simulink model "simulink_model_pid_controller_IT2_controller_ds"  (R2022b)
settings: Solver=VariableStepAuto  StartTime=0.0  StopTime=1  RelTol=1e-3
libraries: slpidlib x1
settings Model: Creator=giris  LastModifiedBy=giris

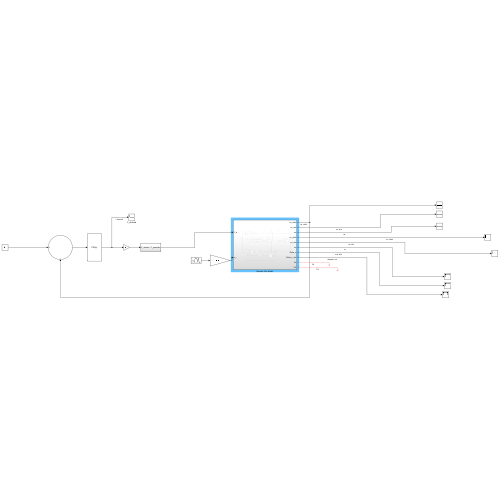
[thumbnail: Simulink's stored preview of the top-level diagram]
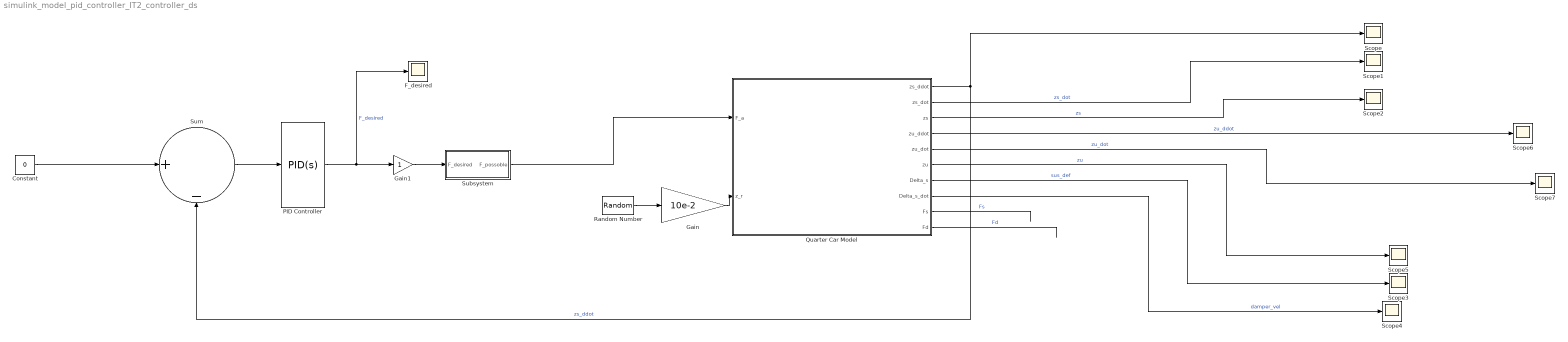
== system simulink_model_pid_controller_IT2_controller_ds ==
  Constant : Constant  Value=0
  F_desired : Scope
  Gain : Gain  Gain=10e-2
  Gain1 : Gain
  PID Controller : slpidlib/PID Controller  Controller=PID  Form=Parallel  TimeDomain=Continuous-time  UseExternalTs=off  SampleTime=-1  IntegratorMethod=Forward Euler  FilterMethod=Forward Euler  ControllerParametersSource=internal  P=8000  I=500  UseKiTs=off  D=400  N=100  UseFilter=on  TunerSelectOption=Transfer Function Based (PID Tuner App)  InitialConditionSource=internal  InitialConditionForIntegrator=0  InitialConditionForFilter=0  DifferentiatorICPrevScaledInput=0  ExternalReset=none  TrackingMode=off  Kt=1  LimitOutput=off  SatLimitsSource=internal  UpperSaturationLimit=inf  LowerSaturationLimit=-inf  LinearizeAsGain=on  AntiWindupMode=none  Kb=1  LimitIntegrator=off  UpperIntegratorSaturationLimit=inf  LowerIntegratorSaturationLimit=-inf  POutMin=[]  POutMax=[]  IOutMin=[]  IOutMax=[]  DOutMin=[]  DOutMax=[]  NOutMin=[]  NOutMax=[]  SumOutMin=[]  SumOutMax=[]  SaturationOutMin=[]  SaturationOutMax=[]  PParamMin=[]  PParamMax=[]  IParamMin=[]  IParamMax=[]  DParamMin=[]  DParamMax=[]  NParamMin=[]  NParamMax=[]  KbParamMin=[]  KbParamMax=[]  KtParamMin=[]  KtParamMax=[]  KbOutMin=[]  KbOutMax=[]  KtOutMin=[]  KtOutMax=[]  IntegratorOutMin=[]  IntegratorOutMax=[]  FilterOutMin=[]  FilterOutMax=[]  SumI1OutMin=[]  SumI1OutMax=[]  SumI2OutMin=[]  SumI2OutMax=[]  SumI3OutMin=[]  SumI3OutMax=[]  SumI4OutMin=[]  SumI4OutMax=[]  SumDOutMin=[]  SumDOutMax=[]  DifferentiatorOutMin=[]  DifferentiatorOutMax=[]  FilterDiffOutCoefMin=[]  FilterDiffOutCoefMax=[]  ReciprocalOutMin=[]  ReciprocalOutMax=[]  SumDenOutMin=[]  SumDenOutMax=[]  SumNumOutMin=[]  SumNumOutMax=[]  DivideOutMin=[]  DivideOutMax=[]  UdiffTsProdOutMin=[]  UdiffTsProdOutMax=[]  NTsProdOutMin=[]  NTsProdOutMax=[]  UintegralTsProdOutMin=[]  UintegralTsProdOutMax=[]  UngainTsProdOutMin=[]  UngainTsProdOutMax=[]  ClampingZeroOutDataTypeStr=Inherit: Inherit via back propagation  ClampingZeroOutMin=[]  ClampingZeroOutMax=[]  FilterDenConstantOutDataTypeStr=Inherit: Inherit via back propagation  FilterDenConstantOutMin=[]  FilterDenConstantOutMax=[]  PCopyOutDataTypeStr=Inherit: Inherit via back propagation  PCopyOutMin=[]  PCopyOutMax=[]  NCopyOutDataTypeStr=Inherit: Inherit via back propagation  NCopyOutMin=[]  NCopyOutMax=[]  IntegratorContinuousStateAttributes=''  IntegratorStateMustResolveToSignalObject=off  IntegratorRTWStateStorageClass=Auto  FilterContinuousStateAttributes=''  FilterStateMustResolveToSignalObject=off  FilterRTWStateStorageClass=Auto  ParallelPVariant=InternalParameters  IdealPVariant=Disabled  IVariant=InternalParameters  DVariant=InternalParameters  IntegratorVariant=Continuous  SatVariant=Disabled  AWVariant=Passthrough  PCopyVariant=Disabled  TRVariant=Disabled  FdbkBlocksVariant=Forward  IdealPFdbkVariant=Disabled  SatFdbkVariant=Disabled  DerivativeFilterVariant=ContFilter  NVariant=InternalParameters  NCopyVariant=Disabled  FilterICVariant=InternalICsFilter  IntegratorICVariant=InternalICs  ExternalResetVariant=Disabled  TRSumVariant=Passthrough  SumFdbkVariant=Disabled  SumVariant=Sum_PID  TsampFilterVariant=InternalTs  TsampNgainVariant=Passthrough  TsampIntegralVariant=Passthrough  ExternalSaturationOutDataTypeStr=Inherit: Same as second input
  Quarter Car Model : Subsystem
  Random Number : RandomNumber  SampleTime=0.01
  Scope{,1..7} (8 alike) : Scope
  Subsystem : Subsystem
  Sum : Sum  Inputs=|+-
  wires:
  PID Controller/1 -> F_desired/1, Gain1/1  "F_desired"
  Random Number/1 -> Gain/1
  Gain/1 -> Quarter Car Model/2(z_r)
  Quarter Car Model/1(zs_ddot) -> Sum/2, Scope/1  "zs_ddot"
  Quarter Car Model/2(zs_dot) -> Scope1/1  "zs_dot"
  Quarter Car Model/3(zs) -> Scope2/1  "zs"
  Constant/1 -> Sum/1
  Sum/1 -> PID Controller/1
  Subsystem/1(F_possoble) -> Quarter Car Model/1(F_a)
  Quarter Car Model/7(Delta_s) -> Scope3/1  "sus_def"
  Quarter Car Model/8(Delta_s_dot) -> Scope4/1  "damper_vel"
  Quarter Car Model/6(zu) -> Scope5/1  "zu"
  Quarter Car Model/4(zu_ddot) -> Scope6/1  "zu_ddot"
  Quarter Car Model/5(zu_dot) -> Scope7/1  "zu_dot"
  Quarter Car Model/9(Fs) -> ?  "Fs"
  Quarter Car Model/10(Fd) -> ?  "Fd"
  Gain1/1 -> Subsystem/1(F_desired)

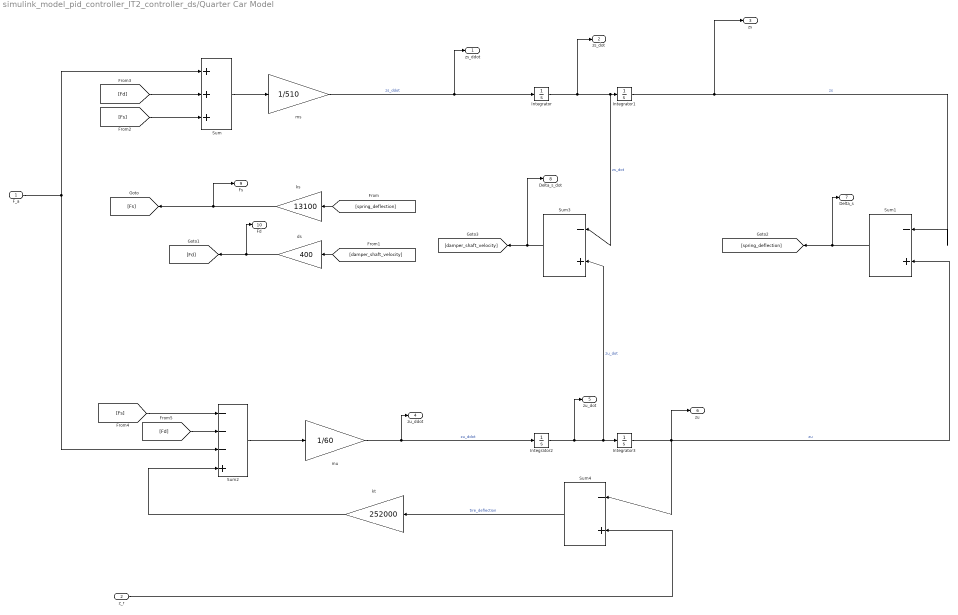
== system simulink_model_pid_controller_IT2_controller_ds/Quarter Car Model ==
  F_a : Inport
  z_r : Inport  Port=2
  Integrator{,1..3} (4 alike) : Integrator
  Sum : Sum  Inputs=+++
  Sum1 : Sum  Inputs=|-+
  Sum2 : Sum  Inputs=---+
  Sum3 : Sum  Inputs=|-+
  Sum4 : Sum  Inputs=|-+
  ds : Gain  Gain=400
  ks : Gain  Gain=13100
  kt : Gain  Gain=252000
  ms : Gain  Gain=1/510
  mu : Gain  Gain=1/60
  zs_ddot : Outport
  zs_dot : Outport  Port=2
  zs : Outport  Port=3
  zu_ddot : Outport  Port=4
  zu_dot : Outport  Port=5
  zu : Outport  Port=6
  Delta_s : Outport  Port=7
  Delta_s_dot : Outport  Port=8
  Fs : Outport  Port=9
  Fd : Outport  Port=10
  wires:
  [spring_deflection] -> ks/1
  [damper_shaft_velocity] -> ds/1
  Integrator/1 -> zs_dot/1, Sum3/1, Integrator1/1  "zs_dot"
  Integrator1/1 -> zs/1, Sum1/1  "zs"
  Sum/1 -> ms/1
  [Fs] -> Sum/3
  ks/1 -> Fs/1, [Fs]
  ds/1 -> Fd/1, [Fd]
  [Fd] -> Sum/2
  F_a/1 -> Sum/1, Sum2/3
  Sum1/1 -> Delta_s/1, [spring_deflection]
  [Fs] -> Sum2/1
  [Fd] -> Sum2/2
  Sum2/1 -> mu/1
  Integrator2/1 -> zu_dot/1, Sum3/2, Integrator3/1  "zu_dot"
  Integrator3/1 -> Sum4/1, Sum1/2, zu/1  "zu"
  Sum3/1 -> Delta_s_dot/1, [damper_shaft_velocity]
  kt/1 -> Sum2/4
  Sum4/1 -> kt/1  "tire_deflection"
  z_r/1 -> Sum4/2
  ms/1 -> zs_ddot/1, Integrator/1  "zs_ddot"
  mu/1 -> zu_ddot/1, Integrator2/1  "zu_ddot"

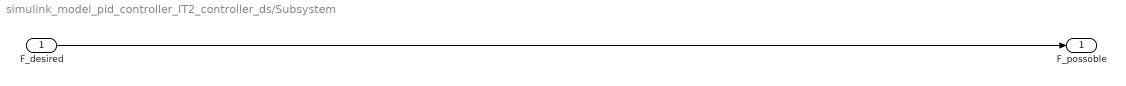
== system simulink_model_pid_controller_IT2_controller_ds/Subsystem ==
  F_desired : Inport
  F_possoble : Outport
  wires:
  F_desired/1 -> F_possoble/1
